simulink model "Online_Ordering_System_Activity_Diagram"  (R2024a)
settings: Solver=VariableStepAuto  StartTime=0.0  StopTime=10.0  RelTol=1e-3
(part 2 of 2)

== system Online_Ordering_System_Activity_Diagram/Display Payment Confirmation Interface ==
  InputPin : Inport
  OutputPin : Outport  OutDataTypeStr=double  PortDimensions=1

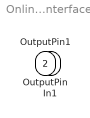
== system Online_Ordering_System_Activity_Diagram/Display Review Order Interface ==
  In1 : Inport
  OutputPin : Outport  OutDataTypeStr=double  PortDimensions=1
  OutputPin1 : Outport  Port=2  OutDataTypeStr=double  PortDimensions=1

== system Online_Ordering_System_Activity_Diagram/Display Search Result ==
  InputPin : Inport
  Out1 : Outport

== system Online_Ordering_System_Activity_Diagram/Enter // Edit Product  Menu ==
  InputPin : Inport
  Out1 : Outport

== system Online_Ordering_System_Activity_Diagram/Enter // Edit Product  Price ==
  In1 : Inport
  Out1 : Outport

== system Online_Ordering_System_Activity_Diagram/Enter // Edit Product Description ==
  In1 : Inport
  Out1 : Outport

== system Online_Ordering_System_Activity_Diagram/Enter // Edit Product Images ==
  In1 : Inport
  Out1 : Outport

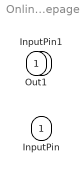
== system Online_Ordering_System_Activity_Diagram/Homepage ==
  InputPin : Inport
  InputPin1 : Inport  Port=2
  Out1 : Outport

== system Online_Ordering_System_Activity_Diagram/Initial ==
  Out1 : Outport

== system Online_Ordering_System_Activity_Diagram/Initial1 ==
  Out1 : Outport

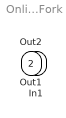
== system Online_Ordering_System_Activity_Diagram/JoinFork ==
  In1 : Inport
  Out1 : Outport
  Out2 : Outport  Port=2

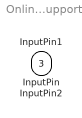
== system Online_Ordering_System_Activity_Diagram/Live Customer Support ==
  InputPin : Inport
  InputPin1 : Inport  Port=2
  InputPin2 : Inport  Port=3

== system Online_Ordering_System_Activity_Diagram/Manage Customer Account Settings ==
  InputPin : Inport
  OutputPin : Outport  OutDataTypeStr=double  PortDimensions=1
  OutputPin1 : Outport  Port=2  OutDataTypeStr=double  PortDimensions=1

== system Online_Ordering_System_Activity_Diagram/Manage Merchant Account Settings ==
  InputPin : Inport
  OutputPin : Outport  OutDataTypeStr=double  PortDimensions=1
  OutputPin2 : Outport  Port=2  OutDataTypeStr=double  PortDimensions=1

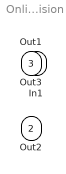
== system Online_Ordering_System_Activity_Diagram/MergeDecision ==
  In1 : Inport
  Out3 : Outport
  Out2 : Outport  Port=2
  Out1 : Outport  Port=3

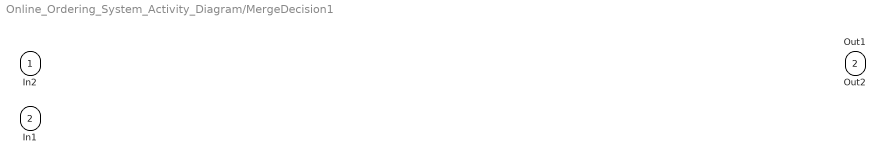
== system Online_Ordering_System_Activity_Diagram/MergeDecision1 ==
  In2 : Inport
  In1 : Inport  Port=2
  Out2 : Outport
  Out1 : Outport  Port=2

== system Online_Ordering_System_Activity_Diagram/MergeDecision10 ==
  In1 : Inport
  Out2 : Outport
  Out1 : Outport  Port=2

== system Online_Ordering_System_Activity_Diagram/MergeDecision11 ==
  In1 : Inport
  Out2 : Outport
  Out1 : Outport  Port=2

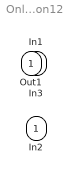
== system Online_Ordering_System_Activity_Diagram/MergeDecision12 ==
  In2 : Inport
  In1 : Inport  Port=2
  In3 : Inport  Port=3
  Out1 : Outport

== system Online_Ordering_System_Activity_Diagram/MergeDecision2 ==
  In2 : Inport
  In1 : Inport  Port=2
  Out1 : Outport

== system Online_Ordering_System_Activity_Diagram/MergeDecision3 ==
  In1 : Inport
  In2 : Inport  Port=2
  Out1 : Outport

== system Online_Ordering_System_Activity_Diagram/MergeDecision4 ==
  In1 : Inport
  Out2 : Outport
  Out1 : Outport  Port=2

== system Online_Ordering_System_Activity_Diagram/MergeDecision5 ==
  In1 : Inport
  Out1 : Outport
  Out2 : Outport  Port=2

== system Online_Ordering_System_Activity_Diagram/MergeDecision6 ==
  In1 : Inport
  In2 : Inport  Port=2
  Out1 : Outport

== system Online_Ordering_System_Activity_Diagram/MergeDecision7 ==
  In1 : Inport
  Out2 : Outport
  Out1 : Outport  Port=2

== system Online_Ordering_System_Activity_Diagram/MergeDecision8 ==
  In1 : Inport
  In2 : Inport  Port=2
  Out1 : Outport

== system Online_Ordering_System_Activity_Diagram/MergeDecision9 ==
  In1 : Inport
  Out2 : Outport
  Out1 : Outport  Port=2

== system Online_Ordering_System_Activity_Diagram/Not Enough Money // Don't Need Product Anymore ==
  In1 : Inport

== system Online_Ordering_System_Activity_Diagram/Order Finished ==
  In2 : Inport
  In1 : Inport  Port=2

== system Online_Ordering_System_Activity_Diagram/Process Gift Card Payment ==
  In1 : Inport
  OutputPin : Outport  OutDataTypeStr=double  PortDimensions=1

== system Online_Ordering_System_Activity_Diagram/Process Online Payment Using CC // DC // Paypal  // Venmo // Alipay ==
  In1 : Inport
  OutputPin : Outport  OutDataTypeStr=double  PortDimensions=1

== system Online_Ordering_System_Activity_Diagram/Prompt Discounts & Rewords ==
  In1 : Inport
  OutputPin1 : Outport  OutDataTypeStr=double  PortDimensions=1
  OutputPin : Outport  Port=2  OutDataTypeStr=double  PortDimensions=1

== system Online_Ordering_System_Activity_Diagram/Prompt GPS Tracking Function ==
  InputPin : Inport
  Out1 : Outport

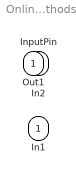
== system Online_Ordering_System_Activity_Diagram/Prompt Payment Methods ==
  In1 : Inport
  InputPin : Inport  Port=2
  In2 : Inport  Port=3
  Out1 : Outport

== system Online_Ordering_System_Activity_Diagram/Quit App ==
  In1 : Inport

== system Online_Ordering_System_Activity_Diagram/Remove Products ==
  In1 : Inport
  Out1 : Outport

== system Online_Ordering_System_Activity_Diagram/Searching Shop // Product ==
  In1 : Inport
  OutputPin : Outport  OutDataTypeStr=double  PortDimensions=1

== system Online_Ordering_System_Activity_Diagram/Send Discount Notification ==
  InputPin : Inport
  InputPin1 : Inport  Port=2

== system Online_Ordering_System_Activity_Diagram/Show Invalid Login // Password ==
  In2 : Inport
  Out1 : Outport

== system Online_Ordering_System_Activity_Diagram/Show Login Successful ==
  In1 : Inport
  OutputPin : Outport  OutDataTypeStr=double  PortDimensions=1

== system Online_Ordering_System_Activity_Diagram/Sign User In ==
  InputPin : Inport
  OutputPin : Outport  OutDataTypeStr=double  PortDimensions=1

== system Online_Ordering_System_Activity_Diagram/User Enters Account Name & Password ==
  InputPin1 : Inport
  In2 : Inport  Port=2
  Out1 : Outport

== system Online_Ordering_System_Activity_Diagram/View Shopping Cart ==
  In1 : Inport
  Out1 : Outport

== system Online_Ordering_System_Activity_Diagram/[else] ==
  In1 : Inport
  Out1 : Outport
  Out2 : Outport  Port=2

== system Online_Ordering_System_Activity_Diagram/[else]1 ==
  In1 : Inport
  Out1 : Outport
  Out2 : Outport  Port=2

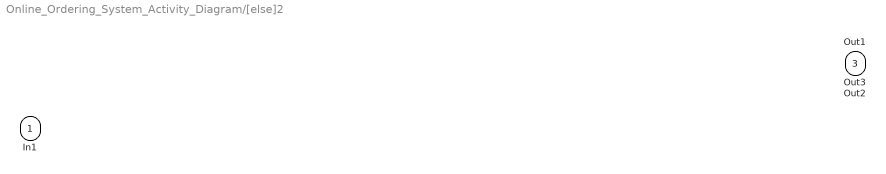
== system Online_Ordering_System_Activity_Diagram/[else]2 ==
  In1 : Inport
  Out3 : Outport
  Out1 : Outport  Port=2
  Out2 : Outport  Port=3
